simulink model "PID_dsp48"  (R2013b)
settings: Solver=ode45  StartTime=0.0  StopTime=10.0  RelTol=1e-3
undefined symbols (not defined in the file): A, A2, B, D, X, Z
libraries: xbsIndex_r4 x15
settings Model: Creator=Gert-Jan  LastModifiedBy=Gert-Jan
settings DebuggingCC: SingleTaskRateTransMsg=error

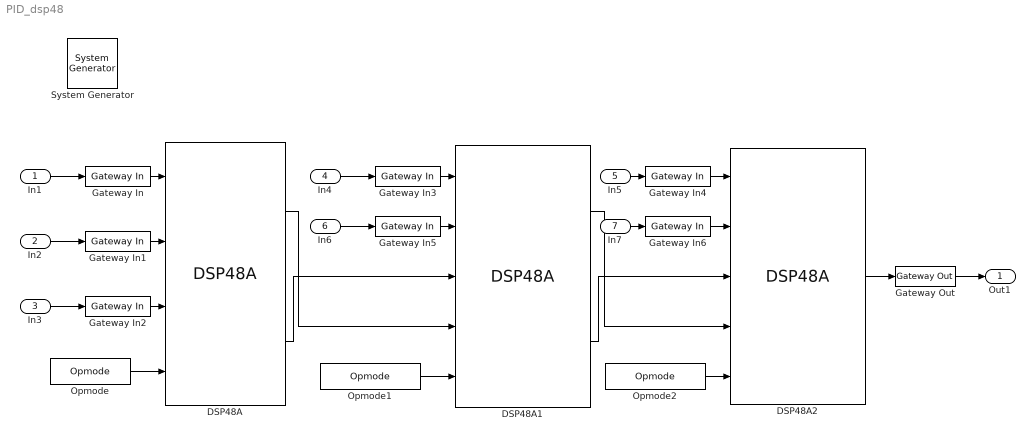
== system PID_dsp48 ==
  In1 : Inport
  In2 : Inport  Port=2
  In3 : Inport  Port=3
  In4 : Inport  Port=4
  In5 : Inport  Port=5
  In6 : Inport  Port=6
  In7 : Inport  Port=7
  " System Generator" : xbsIndex_r4/ System Generator  Tag=genX  xilinxfamily=Kintex7  part=xc7k325t  speed=-3  package=fbg676  synthesis_tool=XST  clock_wrapper=Clock Enables  directory=./netlist  proj_type=Project Navigator  Synth_file=XST Defaults  Impl_file=ISE Defaults  testbench=off  simulink_period=1  sysclk_period=10  dcm_input_clock_period=10  incr_netlist=off  trim_vbits=Everywhere in SubSystem  dbl_ovrd=According to Block Masks  core_generation=According to Block Masks  run_coregen=off  deprecated_control=off  eval_field=0  block_type=sysgen
  DSP48A : xbsIndex_r4/DSP48A  use_op=on  use_creg=off  use_d=on  use_pcin=off  use_pcout=off  use_bcout=on  use_carryin=off  use_carryout=off  rst_all=off  en_all=off  carryin_type=Direct from carry in port  use_a0reg=on  use_a1reg=off  use_b0reg=on  use_b1reg=on  pipeline_c=on  pipeline_d=off  pipeline_mult=off  pipeline_p=on  pipeline_opmode=off  pipeline_carryin=on  rst_a=off  rst_b=off  rst_c=off  rst_d=off  rst_mult=off  rst_p=off  rst_opmode=off  rst_carry_in=off  en_a=off  en_b=off  en_c=off  en_d=off  en_mult=off  en_p=off  en_opmode=off  en_carry_in=off  dbl_ovrd=off  use_synth_model=off  device=3  block_type=dsp48a
  DSP48A1 : xbsIndex_r4/DSP48A  use_op=on  use_creg=off  use_d=on  use_pcin=on  use_pcout=off  use_bcout=on  use_carryin=off  use_carryout=off  rst_all=off  en_all=off  carryin_type=Direct from carry in port  use_a0reg=off  use_a1reg=off  use_b0reg=off  use_b1reg=off  pipeline_c=on  pipeline_d=on  pipeline_mult=on  pipeline_p=on  pipeline_opmode=off  pipeline_carryin=on  rst_a=off  rst_b=off  rst_c=off  rst_d=off  rst_mult=off  rst_p=off  rst_opmode=off  rst_carry_in=off  en_a=off  en_b=off  en_c=off  en_d=off  en_mult=off  en_p=off  en_opmode=off  en_carry_in=off  dbl_ovrd=off  use_synth_model=off  device=3  block_type=dsp48a
  DSP48A2 : xbsIndex_r4/DSP48A  use_op=on  use_creg=off  use_d=on  use_pcin=on  use_pcout=off  use_bcout=off  use_carryin=off  use_carryout=off  rst_all=off  en_all=off  carryin_type=Direct from carry in port  use_a0reg=off  use_a1reg=off  use_b0reg=off  use_b1reg=off  pipeline_c=on  pipeline_d=on  pipeline_mult=on  pipeline_p=on  pipeline_opmode=on  pipeline_carryin=on  rst_a=off  rst_b=off  rst_c=off  rst_d=off  rst_mult=off  rst_p=off  rst_opmode=off  rst_carry_in=off  en_a=off  en_b=off  en_c=off  en_d=off  en_mult=off  en_p=off  en_opmode=off  en_carry_in=off  dbl_ovrd=off  use_synth_model=off  device=3  block_type=dsp48a
  Gateway In{,1..6} (7 alike) : xbsIndex_r4/Gateway In  gui_display_data_type=Fixed-point  arith_type="Signed  (2's comp)"  n_bits=18  bin_pt=0  preci_type=Single  exp_width=8  frac_width=24  quantization="Round  (unbiased: +/- Inf)"  overflow=Saturate  period=1  dbl_ovrd=off  timing_constraint=None  locs_specified=off  LOCs={}  UseAsADC=off  ADCChannel='1'  inherit_from_input=off  hdl_port=on  block_type=gatewayin
  Gateway Out : xbsIndex_r4/Gateway Out  inherit_from_input=off  hdl_port=on  timing_constraint=None  locs_specified=off  LOCs={}  UseAsDAC=off  DACChannel='1'  block_type=gatewayout
  Opmode : xbsIndex_r4/Opmode  device=DSP48A  equ=P=+(A*(D-B))  operation=Custom  inmode_0_3=D+A2  inmode_4=B2  logicinstr=X + Z  z_mux=0  operand=+  xy_mux=P  x_mux=A*(D-B)  carry=0  dbl_ovrd=off  block_type=opmode
  Opmode1 : xbsIndex_r4/Opmode  device=DSP48A  equ=P=PCIN+(A*(D+B))  operation=Custom  inmode_0_3=D+A2  inmode_4=B2  logicinstr=X + Z  z_mux=PCIN  operand=+  xy_mux=P  x_mux=A*(D+B)  carry=0  dbl_ovrd=off  block_type=opmode
  Opmode2 : xbsIndex_r4/Opmode  device=DSP48A  equ=P=PCIN+(A*(D+B))  operation=Custom  inmode_0_3=D+A2  inmode_4=B2  logicinstr=X + Z  z_mux=PCIN  operand=+  xy_mux=P  x_mux=A*(D+B)  carry=0  dbl_ovrd=off  block_type=opmode
  Out1 : Outport
  wires:
  DSP48A/2 -> DSP48A1/3
  DSP48A/1 -> DSP48A1/4
  DSP48A1/2 -> DSP48A2/3
  DSP48A1/1 -> DSP48A2/4
  Opmode/1 -> DSP48A/4
  Opmode1/1 -> DSP48A1/5
  Opmode2/1 -> DSP48A2/5
  Gateway In/1 -> DSP48A/1
  Gateway In1/1 -> DSP48A/2
  Gateway In2/1 -> DSP48A/3
  Gateway In3/1 -> DSP48A1/1
  Gateway In4/1 -> DSP48A2/1
  DSP48A2/1 -> Gateway Out/1
  Gateway Out/1 -> Out1/1
  In1/1 -> Gateway In/1
  In2/1 -> Gateway In1/1
  In3/1 -> Gateway In2/1
  In4/1 -> Gateway In3/1
  In5/1 -> Gateway In4/1
  Gateway In6/1 -> DSP48A2/2
  Gateway In5/1 -> DSP48A1/2
  In6/1 -> Gateway In5/1
  In7/1 -> Gateway In6/1
